simulink model "Q3_design"  (R2021a)
settings: Solver=FixedStepAuto  StartTime=0.0  StopTime=100  FixedStep=0.0001  RelTol=1e-3
libraries: cstblocks x4
settings Model: Creator=47845  LastModifiedBy=47845

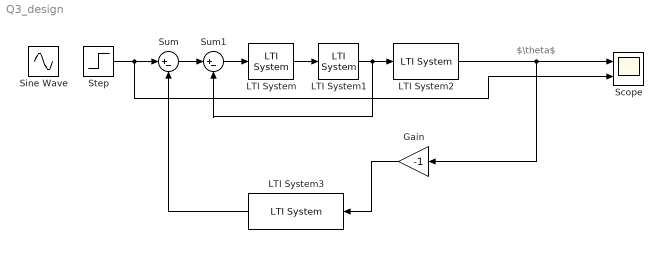
== system Q3_design ==
  note: $\theta$
  Gain : Gain  Gain=-1
  LTI System : cstblocks/LTI System  sys=C  IC=[]
  LTI System1 : cstblocks/LTI System  sys=Py  IC=[]
  LTI System2 : cstblocks/LTI System  sys=Ptheta  IC=[]
  LTI System3 : cstblocks/LTI System  sys=tf(1,[1 1])  IC=[]
  Scope : Scope  NumInputPorts=2
  Sine Wave : Sin  Frequency=10  SampleTime=0
  Step : Step  SampleTime=0
  Sum : Sum  Inputs=|+-
  Sum1 : Sum  Inputs=|+-
  wires:
  Sum1/1 -> LTI System/1
  LTI System/1 -> LTI System1/1
  Step/1 -> Scope/2, Sum/1
  Sum/1 -> Sum1/1
  LTI System1/1 -> Sum1/2, LTI System2/1
  LTI System2/1 -> Gain/1, Scope/1
  LTI System3/1 -> Sum/2
  Gain/1 -> LTI System3/1
